simulink model "V3_sim"  (R2016a)
settings: Solver=VariableStepAuto  StartTime=0.0  StopTime=T_stop  RelTol=1e-3
InitFcn:
  | %V3_initSim
StopFcn:
  | %V3_afterSim
undefined symbols (not defined in the file or in its folder): K, M_AP, stPendel, x0, x_AP
settings Model: Creator=bened  LastModifiedBy=bened
settings GRTTargetCC: GeneratePreprocessorConditionals=Use local settings

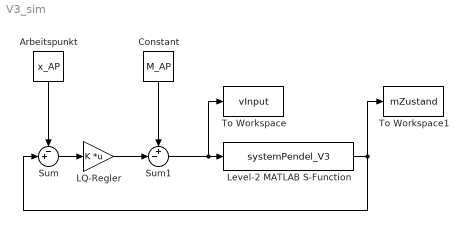
== system V3_sim ==
  Arbeitspunkt : Constant  Value=x_AP
  Constant : Constant  Value=M_AP
  LQ-Regler : Gain  Gain=K  Multiplication=Matrix(K*u)
  Level-2 MATLAB S-Function : M-S-Function  FunctionName=systemPendel_V3  Parameters=stPendel,x0
  Sum : Sum  Inputs=-+|
  Sum1 : Sum  Inputs=+-|
  To Workspace : ToWorkspace  VariableName=vInput  SaveFormat=Structure With Time  SampleTime=-1
  To Workspace1 : ToWorkspace  VariableName=mZustand  SaveFormat=Structure With Time  SampleTime=-1
  wires:
  Level-2 MATLAB S-Function/1 -> Sum/2, To Workspace1/1
  Sum/1 -> LQ-Regler/1
  Arbeitspunkt/1 -> Sum/1
  LQ-Regler/1 -> Sum1/2
  Sum1/1 -> To Workspace/1, Level-2 MATLAB S-Function/1
  Constant/1 -> Sum1/1
